simulink library "Lib"  (R2016b)
settings: Solver=VariableStepAuto  StartTime=0.0  StopTime=10.0  RelTol=1e-3
settings Model: Creator=Odaimoko_  LastModifiedBy=Odaimoko_

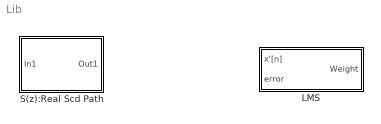
== system Lib ==
  LMS : Subsystem
  S(z):Real Scd Path : Subsystem
      mask Help: S(z):Real Scd Path
      mask Display:
      | port_label('input',1,'In1');
      | port_label('output',1,'Out1');

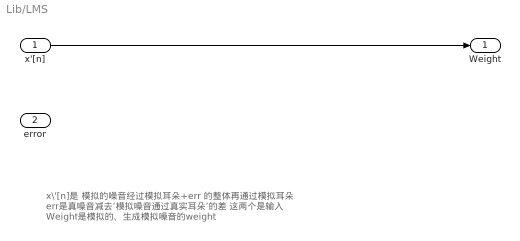
== system Lib/LMS ==
  note: x\'[n]是 模拟的噪音经过模拟耳朵+err 的整体再通过模拟耳朵
      | err是真噪音减去‘模拟噪音通过真实耳朵’的差
      | 这两个是输入
      | Weight是模拟的、生成模拟噪音的weight
  x'[n] : Inport
  error : Inport  Port=2
  Weight : Outport
  wires:
  x'[n]/1 -> Weight/1

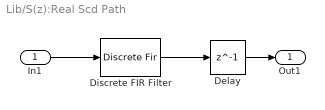
== system Lib/S(z):Real Scd Path ==
  In1 : Inport
  Delay : Delay  DelayLength=1  InitialCondition=0
  Discrete FIR Filter : DiscreteFir  Coefficients=[0.7 0.5 0.5]
  Out1 : Outport
  wires:
  Delay/1 -> Out1/1
  In1/1 -> Discrete FIR Filter/1
  Discrete FIR Filter/1 -> Delay/1
